simulink model "dspwwv"  (Simulink 6.0)
settings: Solver=FixedStepDiscrete  SolverMode=SingleTasking  StartTime=0.0  StopTime=67  RelTol=1e-3  AbsTol=1e-6
undefined symbols (not defined in the file or in its folder): b, magnitude, Ts
libraries: dspsigops x8, dspsrcs4 x5, dspswit3 x5, dspsigattribs x4, simulink x2, dspmlti3 x2, dspsnks4 x1, dspbuff3 x1, dspstat3 x1, dspindex x1
Description:
  | WWV Digital Time-Code Receiver
settings Model: CovMetricSettings=d  Creator=Don Orofino  LastModifiedBy=sconahan  ModifiedHistory=Initial Revision  ExtModeTrigMode=oneshot  ExtModeArmWhenConnect=off  ExtModeAutoUpdateStatusClock=off  ProdHWDeviceType=Specified
settings DataIOCC: SaveOutput=off  SaveTime=off  SignalLoggingName=sigsOut
settings OptimizationCC: InlineInvariantSignals=off  RollThreshold=2
settings DebuggingCC: AlgebraicLoopMsg=error  CheckExecutionContextPreStartOutputMsg=on  CheckExecutionContextRuntimeOutputMsg=on  SolverPrmCheckMsg=none  IntegerOverflowMsg=none  UnconnectedOutputMsg=none
settings HardwareCC: ProdHWDeviceType=Specified
settings RTWCC: GenCodeOnly=on  RTWVerbose=off
settings SFSimCC: SFSimApplyToAllLibs=on  SFSimBuildMode=Incremental

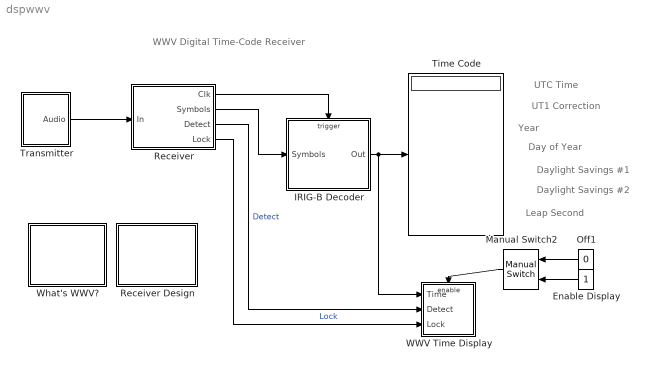
== system dspwwv ==
  note: UTC Time
  note: UT1 Correction
  note: Year
  note: Day of Year
  note: Daylight Savings #1
  note: Daylight Savings #2
  note: Leap Second
  note: WWV Digital Time-Code Receiver
  Enable Display : Constant  Orientation=left  OutDataTypeMode=boolean
  IRIG-B Decoder : Subsystem  TreatAsAtomicUnit=on  PropExecContextAcrossSSBoundary=on
  Manual Switch2 : simulink/Signal Routing/Manual Switch  Orientation=left  sw=1  action=0
  Off1 : Constant  Orientation=left  Value=0  OutDataTypeMode=boolean
  Receiver : Subsystem  PropExecContextAcrossSSBoundary=on
  Receiver Design : Subsystem  PropExecContextAcrossSSBoundary=on
      mask Type: WWV Info
      mask Display: disp('Receiver\nDesign')
  Time Code : Display
  Transmitter : Subsystem  PropExecContextAcrossSSBoundary=on
  WWV Time Display : Subsystem  TreatAsAtomicUnit=on  PropExecContextAcrossSSBoundary=on  mask(WWV Time Display){FigPos=[50 50 230 230]}
      mask prompts: FigPos "Figure position:"
      mask help: Display WWV time-code data in a Handle Graphics window.
      mask init:
      | s.FigPos = FigPos;
      settings: CopyFcn=sdspwwvdisp([],[],[],'BlockCopy');  DeleteFcn=sdspwwvdisp([],[],[],'BlockDelete');  NameChangeFcn=sdspwwvdisp([],[],[],'NameChange');
      mask Help: Display WWV time-code data in a Handle Graphics window.
      mask Display: disp('WWV\nDisplay')
  What's WWV? : Subsystem  PropExecContextAcrossSSBoundary=on
      mask Type: WWV Info
      mask Display: disp('What''s\nWWV?')
  wires:
  Receiver/2(Symbols) -> IRIG-B Decoder/1(Symbols)
  IRIG-B Decoder/1(Out) -> Time Code/1, WWV Time Display/1(Time)
  Receiver/1(Clk) -> IRIG-B Decoder/Trigger
  Transmitter/1(Audio) -> Receiver/1(In)
  Receiver/4(Lock) -> WWV Time Display/3(Lock)  "Lock"
  Receiver/3(Detect) -> WWV Time Display/2(Detect)  "Detect"
  Off1/1 -> Manual Switch2/1
  Enable Display/1 -> Manual Switch2/2
  Manual Switch2/1 -> WWV Time Display/Enable

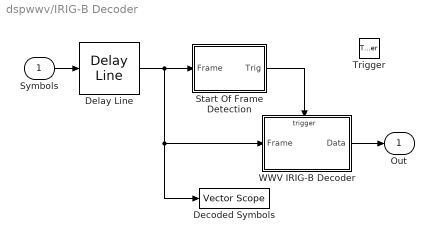
== system dspwwv/IRIG-B Decoder ==
  Symbols : Inport  LatchInput=off
  Trigger : TriggerPort  StatesWhenEnabling=reset
  Decoded Symbols : dspsnks4/Vector Scope  ScopeProperties=on  Domain=User-defined  HorizSpan=1  DisplayProperties=off  AxisGrid=on  Memory=off  FrameNumber=on  AxisLegend=off  AxisZoom=off  OpenScopeAtSimStart=on  OpenScopeImmediately=off  FigPos=[288 87 633 176]  AxisProperties=off  XUnits=Hertz  XRange=[0...Fs/2]  InheritXIncr=off  XIncr=1  XLabel=Samples  YUnits=dB  YLabel=Symbols  LineProperties=off  LineStyles=None|:  LineMarkers=stem|stem  LineColors=[0 0 1]|[0 0 1]
      settings: YMin=0  YMax=3
  Delay Line : dspbuff3/Delay Line  siz=60  ic=0  directfeed=off
  Start Of Frame Detection : Subsystem  PropExecContextAcrossSSBoundary=on
  WWV IRIG-B Decoder : Subsystem  TreatAsAtomicUnit=on  PropExecContextAcrossSSBoundary=on
  Out : Outport
  wires:
  WWV IRIG-B Decoder/1(Data) -> Out/1
  Start Of Frame Detection/1(Trig) -> WWV IRIG-B Decoder/Trigger
  Symbols/1 -> Delay Line/1
  Delay Line/1 -> Start Of Frame Detection/1(Frame), WWV IRIG-B Decoder/1(Frame), Decoded Symbols/1

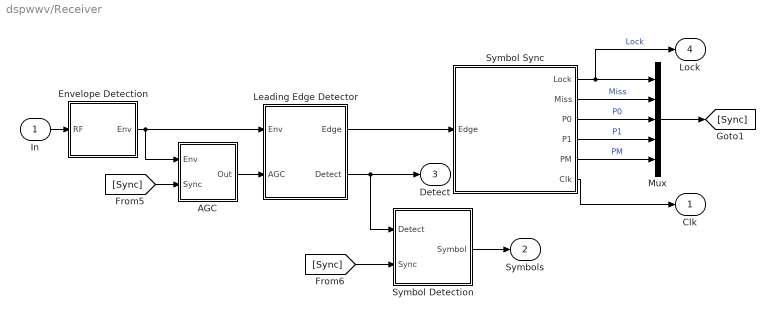
== system dspwwv/Receiver ==
  In : Inport  LatchInput=off
  AGC : Subsystem  PropExecContextAcrossSSBoundary=on
  Envelope Detection : Subsystem  PropExecContextAcrossSSBoundary=on
  Leading Edge Detector : Subsystem  PropExecContextAcrossSSBoundary=on
  Mux : Mux  Inputs=5
  Symbol Detection : Subsystem  PropExecContextAcrossSSBoundary=on
  Symbol Sync : Stateflow chart  PropExecContextAcrossSSBoundary=on
  Clk : Outport  InitialOutput=0
  Symbols : Outport  Port=2  InitialOutput=0
  Detect : Outport  Port=3  InitialOutput=0
  Lock : Outport  Port=4  InitialOutput=0
  wires:
  Envelope Detection/1(Env) -> Leading Edge Detector/1(Env), AGC/1(Env)
  In/1 -> Envelope Detection/1(RF)
  [Sync] -> AGC/2(Sync)
  Leading Edge Detector/2(Detect) -> Symbol Detection/1(Detect), Detect/1
  Symbol Sync/2(Miss) -> Mux/2  "Miss"
  Symbol Sync/5(PM) -> Mux/5  "PM"
  Symbol Sync/6(Clk) -> Clk/1
  [Sync] -> Symbol Detection/2(Sync)
  AGC/1(Out) -> Leading Edge Detector/2(AGC)
  Mux/1 -> [Sync]
  Symbol Sync/3(P0) -> Mux/3  "P0"
  Symbol Sync/4(P1) -> Mux/4  "P1"
  Leading Edge Detector/1(Edge) -> Symbol Sync/1(Edge)
  Symbol Detection/1(Symbol) -> Symbols/1
  Symbol Sync/1(Lock) -> Mux/1, Lock/1  "Lock"

== system dspwwv/Receiver Design ==
  note: This receiver design serves as a simple example of how to use:
      |
      | - Simulink
      | - Signal Processing Blockset
      | - Stateflow
      | - Real-Time Workshop
      |
      | together to achieve an incoherent digital receiver.  The
      | example incorporates Stateflow for achieving symbol
      | synchronization.  Therefore, you must have a compatible
      | C compiler and be able to compile MEX from MATLAB.
      |
      | The transmitted symbols, MARKER, ZERO, ONE, and MISS,
      | are mapped to the following integer values:
      |
      | MISS        = 0
      | ZERO      = 1
      | ONE         = 2
      | MARKER  = 3
      |
      | These values are displayed on the "Decoder Symbols" scope.

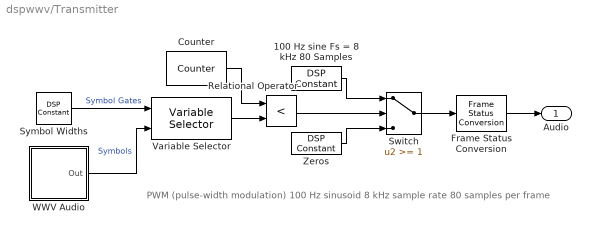
== system dspwwv/Transmitter ==
  note: PWM (pulse-width modulation)
      | 100 Hz sinusoid
      | 8 kHz sample rate
      | 80 samples per frame
  100 Hz sine Fs = 8 kHz 80 Samples : dspsrcs4/DSP Constant  Value=single(sin(2*pi*100*(0:79)/8000))  SampleMode=Continuous  discreteOutput=Sample-based (interpret vectors as 1-D)  continuousOutput=Sample-based (interpret vectors as 1-D)  sampTime=1  framePeriod=1  dataType=Inherit from 'Constant value'  isSigned=on  wordLen=16  udDataType=sfix(16)  fracBitsMode=Best precision  numFracBits=15  InterpretAs1D=on  Ts=1  FramebasedOutput=off
  Counter : dspswit3/Counter  Direction=Up  CountEvent=Free running  CounterSize=User defined  MaxCount=99  InitialCount=0  Output=Count  HitValue=32  ResetInput=off  SamplesPerFrame=1  Ts=1/100  CntDtype=single  HitDtype=Logical
  Frame Status Conversion : dspsigattribs/Frame Status Conversion  growRefPort=off  outframe=Frame-based
  Relational Operator : RelationalOperator  Operator=<  InputSameDT=on
  Switch : Switch  Threshold=1  SaturateOnIntegerOverflow=on  InputSameDT=on
  Symbol Widths : dspsrcs4/DSP Constant  Value=single([0 17 47 77])  SampleMode=Discrete  discreteOutput=Sample-based (interpret vectors as 1-D)  continuousOutput=Sample-based  sampTime=1  framePeriod=2  dataType=Inherit from 'Constant value'  isSigned=on  wordLen=16  udDataType=sfix(16)  fracBitsMode=Best precision  numFracBits=15  InterpretAs1D=-inf  Ts=-inf  FramebasedOutput=-inf
  Variable Selector : dspindex/Variable Selector  rowsOrCols=Rows  IdxMode=Variable  Elements=[1 3]  ZerOneIdxMode=Zero-based  errmode=Clip and Warn
  WWV Audio : Subsystem  PropExecContextAcrossSSBoundary=on  mask(WWV Audio Synthesizer){outp=Symbols, utc=12.34, ut1=+0.2, day=336, yr=2002, dst=off, dst2=off, leap=on, bufsize=1}
      mask prompts: outp "Output:"; utc "Time (hh.mm):"; ut1 "UT1 Correction ([-0.7, +0.7]):"; day "Day of year:"; yr "Year:"; dst "Daylight Savings"; dst2 "Daylight Savings #2"; leap "Leap second"; bufsize "Samples per frame:"
      mask help: Generate 8 kHz sampled test data in WWV IRIG format.
      mask init:
      | s.utc=utc;s.ut1=ut1;s.day=day;s.yr=yr;
      | s.dst=dst;s.dst2=dst2;s.leap=leap; s.mode=outp;
      | [b,Ts]=dspwwvgen(s);
      | 
      | if strcmp(outp,'Audio'),
      | 
      | x = [.1 .2 .2 .1 .1 NaN .2 .35 .35 .2 .2 NaN .35 .4 .4 .35 .35];
      | y = [.4 .4 .6 .6 .4 NaN .4 .1  .9  .6 .4 NaN .1  .1 .9 .9  .1 ];
      | a=.5;  s=5*pi/180;  t = -s:pi/180:s; x = [x NaN a*cos(t)]; y = [y NaN a*sin(t)+.5];
      | a=.65; s=10*pi/180; t = -s:pi/180:s; x = [x NaN a*cos(t)]; y = [y NaN a*sin(t)+.5];
      | a=.8;  s=20*pi/180; t = -s:pi/180:s; x = [x NaN a*cos(t)]; y = [y NaN a*sin(t)+.5];
      | 
      | else
      | x = [.1 .2 .2 .3 .3 .5 .5 .8 .8 .9];
      | y = [.2 .2 .8 .8 .2 .2 .8 .8 .2 .2];
      | end
      mask Help: Generate 8 kHz sampled test data in WWV IRIG format.
      mask StyleString: popup(Symbols|Audio),edit,edit,edit,edit,checkbox,checkbox,checkbox,edit
      mask Display: plot(x,y)
  Zeros : dspsrcs4/DSP Constant  Value=single(zeros(80,1))  SampleMode=Continuous  discreteOutput=Sample-based (interpret vectors as 1-D)  continuousOutput=Sample-based (interpret vectors as 1-D)  sampTime=1  framePeriod=1  dataType=Inherit from 'Constant value'  isSigned=on  wordLen=16  udDataType=sfix(16)  fracBitsMode=Best precision  numFracBits=15  InterpretAs1D=on  Ts=1  FramebasedOutput=off
  Audio : Outport
  wires:
  100 Hz sine Fs = 8 kHz 80 Samples/1 -> Switch/1
  Zeros/1 -> Switch/3
  Switch/1 -> Frame Status Conversion/1
  WWV Audio/1(Out) -> Variable Selector/2  "Symbols"
  Symbol Widths/1 -> Variable Selector/1  "Symbol Gates"
  Frame Status Conversion/1 -> Audio/1
  Counter/1 -> Relational Operator/1
  Relational Operator/1 -> Switch/2
  Variable Selector/1 -> Relational Operator/2

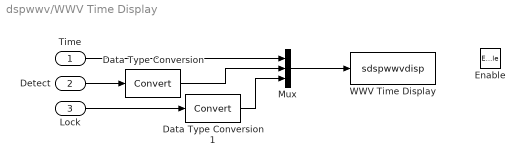
== system dspwwv/WWV Time Display ==
  Time : Inport  LatchInput=off
  Detect : Inport  Port=2  LatchInput=off
  Lock : Inport  Port=3  LatchInput=off
  Enable : EnablePort
  Data Type Conversion : DataTypeConversion  SaturateOnIntegerOverflow=on  RndMeth=Zero
  Data Type Conversion1 : DataTypeConversion  SaturateOnIntegerOverflow=on  RndMeth=Zero
  Mux : Mux  Inputs=3
  WWV Time Display : S-Function  FunctionName=sdspwwvdisp  Parameters=s
  wires:
  Mux/1 -> WWV Time Display/1
  Detect/1 -> Data Type Conversion/1
  Lock/1 -> Data Type Conversion1/1
  Time/1 -> Mux/1
  Data Type Conversion/1 -> Mux/2
  Data Type Conversion1/1 -> Mux/3

== system dspwwv/What's WWV? ==
  note: WWV is the callsign of a US Government radio station run
      | by the National Institute of Standards and Techology (NIST) in
      | Ft. Collins, Colorado.  It is transmitted on 2.5, 5, 10, 15, and 20 MHz.
      |
      | WWV transmits frequency reference standards and time code
      | information referenced to a Cesium clock, giving a transmission
      | accuracy of 1 part in 100 billion for frequency or 10 uS for timing.
      |
      | The time code is transmitted as a frame of 60 symbols, one symbol
      | per second.  Thus, it takes one minute to transmit a full frame of
      | information.  Each symbol is represented using pulse-width modulation
      | of a 100 Hz audio tone.  There are 3 symbols transmitted: a MARKER
      | symbol (transmitted once every 10 seconds), a ZERO symbol, and a
      | ONE symbol.   Additionally, there is a MISSING symbol transmitted
      | near the start of a frame of data.
      |
      | Time code information includes:
      | - 24 hour time (UTC)
      | - Year
      | - Day of year
      | - Daylight Savings Indicators
      | - Leap Seconds Correction
      | - UT1 time correction

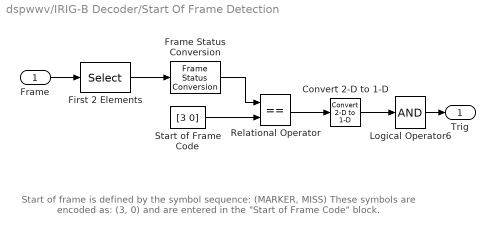
== system dspwwv/IRIG-B Decoder/Start Of Frame Detection ==
  note: Start of frame is defined by the symbol sequence:
      | (MARKER, MISS)
      | These symbols are encoded as:
      | (3, 0)
      | and are entered in the "Start of Frame Code" block.
  Frame : Inport  LatchInput=off
  Convert 2-D to 1-D : dspsigattribs/Convert 2-D to 1-D
  First 2 Elements : Selector  Elements=[1 2]  InputPortWidth=60
  Frame Status Conversion : dspsigattribs/Frame Status Conversion  growRefPort=off  outframe=Sample-based
  Logical Operator6 : Logic  Inputs=1
  Relational Operator : RelationalOperator  Operator===  InputSameDT=on
  Start of Frame Code : Constant  Value=[3 0]  OutDataTypeMode=int8
  Trig : Outport  InitialOutput=0
  wires:
  Start of Frame Code/1 -> Relational Operator/2
  Relational Operator/1 -> Convert 2-D to 1-D/1
  Logical Operator6/1 -> Trig/1
  Frame/1 -> First 2 Elements/1
  First 2 Elements/1 -> Frame Status Conversion/1
  Frame Status Conversion/1 -> Relational Operator/1
  Convert 2-D to 1-D/1 -> Logical Operator6/1

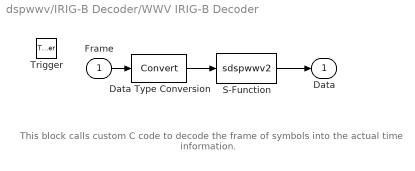
== system dspwwv/IRIG-B Decoder/WWV IRIG-B Decoder ==
  note: This block calls custom C code to decode the
      | frame of symbols into the actual time information.
  Frame : Inport  LatchInput=off
  Trigger : TriggerPort  StatesWhenEnabling=reset
  Data Type Conversion : DataTypeConversion  SaturateOnIntegerOverflow=on  RndMeth=Zero
  S-Function : S-Function  FunctionName=sdspwwv2  Parameters=2000
  Data : Outport  InitialOutput=0
  wires:
  Frame/1 -> Data Type Conversion/1
  S-Function/1 -> Data/1
  Data Type Conversion/1 -> S-Function/1

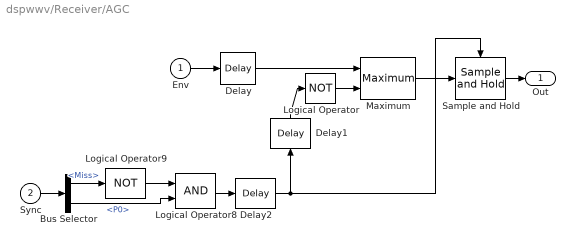
== system dspwwv/Receiver/AGC ==
  Env : Inport  LatchInput=off
  Sync : Inport  Port=2  LatchInput=off
  Bus Selector : BusSelector  DialogController=Simulink.DDGSource_Bus  OutputSignals=Miss,P0
  Delay : dspsigops/Delay  dly_unit=Samples  delay=3  ic_detail=off  dif_ic_for_ch=off  dif_ic_for_dly=off  ic=0  reset_popup=None
  Delay1 : dspsigops/Delay  Orientation=up  dly_unit=Samples  delay=1  ic_detail=off  dif_ic_for_ch=off  dif_ic_for_dly=off  ic=0  reset_popup=None
  Delay2 : dspsigops/Delay  dly_unit=Samples  delay=1  ic_detail=off  dif_ic_for_ch=off  dif_ic_for_dly=off  ic=0  reset_popup=None
  Logical Operator : Logic  Operator=NOT  Inputs=1
  Logical Operator8 : Logic
  Logical Operator9 : Logic  Operator=NOT  Inputs=1
  Maximum : dspstat3/Maximum  DialogController=dspDDGCreate  DialogControllerArgs=DataTag0  fcn=Running  reset=Non-zero sample  roundingMode=Floor  overflowMode=off
  Sample and Hold : dspsigops/Sample and Hold  trig=Falling edge  initCond=single(0.075)
  Out : Outport
  wires:
  Logical Operator9/1 -> Logical Operator8/1
  Bus Selector/2 -> Logical Operator8/2  "<P0>"
  Logical Operator8/1 -> Delay2/1
  Delay2/1 -> Sample and Hold/Trigger, Delay1/1
  Maximum/1 -> Sample and Hold/1
  Logical Operator/1 -> Maximum/2
  Delay1/1 -> Logical Operator/1
  Delay/1 -> Maximum/1
  Env/1 -> Delay/1
  Sample and Hold/1 -> Out/1
  Sync/1 -> Bus Selector/1
  Bus Selector/1 -> Logical Operator9/1  "<Miss>"

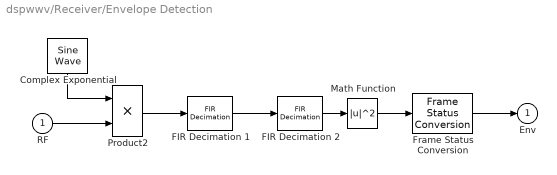
== system dspwwv/Receiver/Envelope Detection ==
  RF : Inport  LatchInput=off
  Complex Exponential : dspsrcs4/Sine Wave  Orientation=down  Amplitude=1  Frequency=100  Phase=0  SampleMode=Discrete  OutComplex=Complex  CompMethod=Table lookup  TableSize=Memory  SampleTime=1/8000  SamplesPerFrame=80  dataType=single  wordLen=16  udDataType=sfix(16)  fracBitsMode=Best precision  numFracBits=14  ResetState=Restart at time zero
      settings: additionalParams=on
  FIR Decimation 1 : dspmlti3/FIR Decimation  DialogController=dspDDGCreate  DialogControllerArgs=DataTag1  h=fir1(31, 1/40)  D=20  framing=Maintain input frame rate  outputBufInitCond=0  roundingMode=Floor  overflowMode=off
  FIR Decimation 2 : dspmlti3/FIR Decimation  DialogController=dspDDGCreate  DialogControllerArgs=DataTag2  h=fir1(15, 1/8)  D=4  framing=Maintain input frame rate  outputBufInitCond=0  roundingMode=Floor  overflowMode=off
  Frame Status Conversion : dspsigattribs/Frame Status Conversion  growRefPort=off  outframe=Sample-based
  Math Function : Math  Operator=magnitude^2  SaturateOnIntegerOverflow=on
  Product2 : Product  SaturateOnIntegerOverflow=on  InputSameDT=on
  Env : Outport  InitialOutput=0
  wires:
  Complex Exponential/1 -> Product2/1
  RF/1 -> Product2/2
  Product2/1 -> FIR Decimation 1/1
  FIR Decimation 1/1 -> FIR Decimation 2/1
  FIR Decimation 2/1 -> Math Function/1
  Math Function/1 -> Frame Status Conversion/1
  Frame Status Conversion/1 -> Env/1

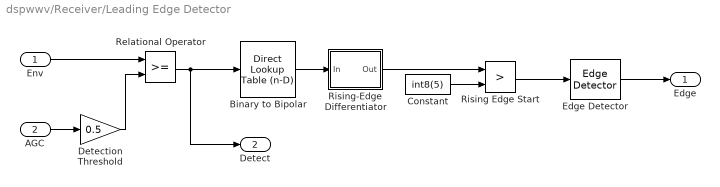
== system dspwwv/Receiver/Leading Edge Detector ==
  Env : Inport  LatchInput=off
  AGC : Inport  Port=2  LatchInput=off
  Binary to Bipolar : simulink/Lookup Tables/Direct Lookup Table (n-D)  maskTabDims=1  explicitNumDims=1  outDims=Element  tabIsInput=off  mxTable=int8([-1, 1])  clipFlag=None
  Constant : Constant  Value=int8(5)
  Detection Threshold : Gain  Gain=0.5  SaturateOnIntegerOverflow=on
  Edge Detector : dspswit3/Edge Detector
  Relational Operator : RelationalOperator  InputSameDT=on
  Rising Edge Start : RelationalOperator  Operator=>  LogicOutDataTypeMode=Boolean  ZeroCross=off
  Rising-Edge Differentiator : Subsystem  PropExecContextAcrossSSBoundary=on
  Edge : Outport  InitialOutput=0
  Detect : Outport  Port=2  InitialOutput=0
  wires:
  AGC/1 -> Detection Threshold/1
  Detection Threshold/1 -> Relational Operator/2
  Relational Operator/1 -> Binary to Bipolar/1, Detect/1
  Edge Detector/1 -> Edge/1
  Rising Edge Start/1 -> Edge Detector/1
  Env/1 -> Relational Operator/1
  Constant/1 -> Rising Edge Start/2
  Binary to Bipolar/1 -> Rising-Edge Differentiator/1(In)
  Rising-Edge Differentiator/1(Out) -> Rising Edge Start/1

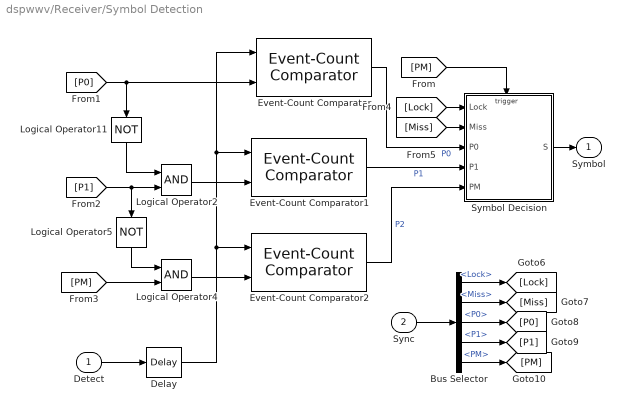
== system dspwwv/Receiver/Symbol Detection ==
  Detect : Inport  LatchInput=off
  Sync : Inport  Port=2  LatchInput=off
  Bus Selector : BusSelector  DialogController=Simulink.DDGSource_Bus  OutputSignals=Lock,Miss,P0,P1,PM
  Delay : dspsigops/Delay  dly_unit=Samples  delay=2  ic_detail=off  dif_ic_for_ch=off  dif_ic_for_dly=off  ic=0  reset_popup=None
  Event-Count Comparator : dspswit3/Event-Count Comparator  Threshold=floor(0.17*50/2)
  Event-Count Comparator1 : dspswit3/Event-Count Comparator  Threshold=floor((0.47-0.17)*50/2)
  Event-Count Comparator2 : dspswit3/Event-Count Comparator  Threshold=floor((0.77-0.47)*50/2)
  Logical Operator11 : Logic  Orientation=down  Operator=NOT  Inputs=1
  Logical Operator2 : Logic
  Logical Operator4 : Logic
  Logical Operator5 : Logic  Orientation=down  Operator=NOT  Inputs=1
  Symbol Decision : Stateflow chart  PropExecContextAcrossSSBoundary=on
  Symbol : Outport  InitialOutput=0
  wires:
  Logical Operator2/1 -> Event-Count Comparator1/2
  [P0] -> Logical Operator11/1, Event-Count Comparator/2
  [P1] -> Logical Operator2/2, Logical Operator5/1
  Logical Operator5/1 -> Logical Operator4/1
  Logical Operator11/1 -> Logical Operator2/1
  Detect/1 -> Delay/1
  [Miss] -> Symbol Decision/2(Miss)
  Symbol Decision/1(S) -> Symbol/1
  [PM] -> Symbol Decision/Trigger
  Event-Count Comparator/1 -> Symbol Decision/3(P0)  "P0"
  Event-Count Comparator1/1 -> Symbol Decision/4(P1)  "P1"
  Event-Count Comparator2/1 -> Symbol Decision/5(PM)  "P2"
  [PM] -> Logical Operator4/2
  [Lock] -> Symbol Decision/1(Lock)
  Delay/1 -> Event-Count Comparator2/1, Event-Count Comparator1/1, Event-Count Comparator/1
  Logical Operator4/1 -> Event-Count Comparator2/2
  Sync/1 -> Bus Selector/1
  Bus Selector/1 -> [Lock]  "<Lock>"
  Bus Selector/2 -> [Miss]  "<Miss>"
  Bus Selector/3 -> [P0]  "<P0>"
  Bus Selector/4 -> [P1]  "<P1>"
  Bus Selector/5 -> [PM]  "<PM>"

== system dspwwv/Transmitter/WWV Audio ==
  Signal From Workspace1 : dspsrcs4/Signal From Workspace  X=int8(b)  Ts=Ts  nsamps=bufsize  OutputAfterFinalValue=Setting to zero
  Out : Outport  InitialOutput=0
  wires:
  Signal From Workspace1/1 -> Out/1

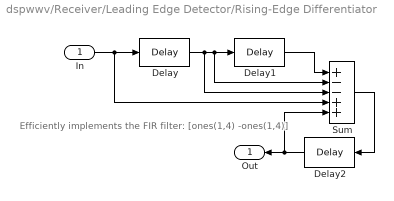
== system dspwwv/Receiver/Leading Edge Detector/Rising-Edge Differentiator ==
  note: Efficiently implements the FIR filter:
      | [ones(1,4) -ones(1,4)]
  In : Inport  LatchInput=off
  Delay : dspsigops/Delay  dly_unit=Samples  delay=4  ic_detail=off  dif_ic_for_ch=off  dif_ic_for_dly=off  ic=0  reset_popup=None
  Delay1 : dspsigops/Delay  dly_unit=Samples  delay=4  ic_detail=off  dif_ic_for_ch=off  dif_ic_for_dly=off  ic=0  reset_popup=None
  Delay2 : dspsigops/Delay  Orientation=left  dly_unit=Samples  delay=1  ic_detail=off  dif_ic_for_ch=off  dif_ic_for_dly=off  ic=0  reset_popup=None
  Sum : Sum  Inputs=+--++  SaturateOnIntegerOverflow=on
  Out : Outport  Orientation=left
  wires:
  In/1 -> Sum/4, Delay/1
  Delay/1 -> Delay1/1, Sum/2, Sum/3
  Sum/1 -> Delay2/1
  Delay2/1 -> Sum/5, Out/1
  Delay1/1 -> Sum/1

== stateflow chart Receiver/Symbol Detection/Symbol Decision ==
  state DecisionLogic() [function]
    (default) -> (junction 5)
    (junction 5) -> (junction 6) : {
        | $ $
        | /* Condition 1: Zero threshold crossed */
        | c1 = (P0);
        | }
    (junction 6) -> (junction 7) : {
        | $ $
        | /* Condition 2: One threshold crossed */
        | c2 = (P1);
        | }
    (junction 7) -> (junction 8) : {
        | $ $
        | /* Condition 3: Marker threshold crossed */
        | c3 = (PM);
        | }
    (junction 8) -> (junction 9) : {
        | $ $
        | /* Condition 4: Is receiver out of lock, or did we miss too many symbols? */
        | c4 = (!Lock  || Miss);
        | }
    (junction 9) -> (junction 10) : [c4]   /* D1 */
    (junction 10) -> (junction 11) : {
        | $ $
        | /* Action 'miss': Missing Symbol Detected */
        | S = 0;
        | }
    (junction 9) -> (junction 12)
    (junction 12) -> (junction 13) : [!c1&&!c2]   /* D2 */
    (junction 13) -> (junction 14) : {
        | $ $
        | /* Action 'miss': Missing Symbol Detected */
        | S = 0;
        | }
    (junction 12) -> (junction 15)
    (junction 15) -> (junction 16) : [c1&&!c2&&!c3]   /* D3 */
    (junction 16) -> (junction 17) : {
        | $ $
        | /* Action 'zero': Zero Symbol Detected */
        | S = 1;
        | }
    (junction 15) -> (junction 18)
    (junction 18) -> (junction 19) : [c2&&!c3]   /* D4 */
    (junction 19) -> (junction 20) : {
        | $ $
        | /* Action 'one': One Symbol Detected */
        | S = 2;
        | }
    (junction 18) -> (junction 21)
    (junction 21) -> (junction 22) : /* Default */
    (junction 22) -> (junction 23) : {
        | $ $
        | /* Action 'mark': Marker Symbol Detected */
        | S = 3;
        | }
  (default) -> (junction 4) : {DecisionLogic();}
  data: c1 temporary boolean; c2 temporary boolean; c3 temporary boolean; c4 temporary boolean; Lock input boolean size=1; Miss input boolean size=1; P0 input boolean size=1; P1 input boolean size=1; PM input boolean size=1; S output int8 size=1
  data c1 settings: description=Zero threshold crossed
  data c2 settings: description=One threshold crossed
  data c3 settings: description=Marker threshold crossed
  data c4 settings: description=Is receiver out of lock, or did we miss too many symbols?
  events: clk input FALLING_EDGE_EVENT

== stateflow chart Receiver/Symbol Sync ==
  settings: sampleTime=0.01
  state Integration [parallel]
    state Running
      Running -> (junction 73) : at(NMarker,tick)
          | {PM=0}
      Running -> (junction 72) : at(NOne,tick)
          | {P1=0;}
      Running -> (junction 74) : at(NZero,tick)
          | {P0=0}
    state Disabled
    Disabled -> Running : tick
    (default) -> Disabled
    Running -> Disabled : en(Sync)
        | {P0=1, P1=1, PM=1}
  state Clock [parallel]
    state ClkLo
    state Clk
    state Rst
    Clk -> ClkLo
    ClkLo -> Clk : every(N1,tick)
        | [ in(Search) ]
    Clock -> Rst : en(Sync)
    (default) -> Rst
    Rst -> Clk
  state SymbolSync [parallel]
    state Search
      state SeekSilence
      state Wait
      state FindPulse
        en: cnt=Nwin
        du: cnt--
      SeekSilence -> SeekSilence : [Edge]
      Wait -> SeekSilence : [Edge]
      SymbolSync.Search.FindPulse -> Wait : [cnt==0]
      SeekSilence -> SymbolSync.Search.FindPulse : after(N1est-Nhalfwin+1,tick)
    state Lock
      state Sync
      state FindPulse
        en: cnt=Nwin
        du: cnt--
      (junction 76) -> Sync : {Miss=1
          | dly=N1-Nwin}
      (junction 75) -> Sync : {Miss = 0
          | N1 += Nhalfwin-cnt
          | dly=N1-Nhalfwin+1}
      Sync -> SymbolSync.Lock.FindPulse : after(dly,tick)
      SymbolSync.Lock.FindPulse -> (junction 75) : [Edge]
      SymbolSync.Lock.FindPulse -> (junction 76) : [cnt==0]
    (default) -> Wait
    (junction 76) -> Wait : [Miss]
    SymbolSync.Search.FindPulse -> (junction 75) : [Edge]
        | {N1=N1est}
  data: NMarker constant int16 size=1 =77; NZero constant int16 size=1 =17; NOne constant int16 size=1 =47; cnt local int16 size=1 [0..127]; N1est constant int16 size=1 =100; Nwin constant int16 size=1 =5; Nhalfwin local int16 size=1 [0..5] =3; dly local int16 size=1; Edge input boolean size=1 [0..1]; Lock output State size=1; Miss output boolean size=1 [0..1]; P0 output boolean size=1 [0..1]; P1 output boolean size=1 [0..1]; PM output boolean size=1 [0..1]; N1 local int16 size=1 [0..1023] =100; Clk output State size=1
  data NMarker settings: description=Number of samples in bit-integration window
  data NZero settings: description=Number of samples in ZERO bit (AGC) integration window
  data N1est settings: description=Esimated of number of samples per bit interval (1 second, i.e., 50 for 50Hz nominal sample frequency)
  data Nwin settings: description=Track window, in samples
  data Nhalfwin settings: description=Half of Nwin, (Nwin+1)/2
  data N1 settings: description=Number of samples per bit interval (1 second), corrected during track
